simulink model "CTDSM_CIFF_OPAMP_NESTED_CHOPPING"  (R2025b)
settings: Solver=VariableStepAuto  StartTime=0.0  StopTime=0.5  RelTol=1e-3
libraries: fl_lib x19, nesl_utility x8, ee_lib x4, simulink_extras x1, cstblocks x1, dspobslib x1
settings Model: Creator=Hp  LastModifiedBy=k2vas

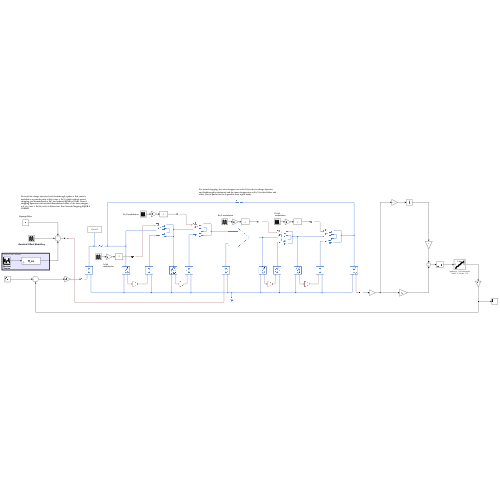
[thumbnail: Simulink's stored preview of the top-level diagram]
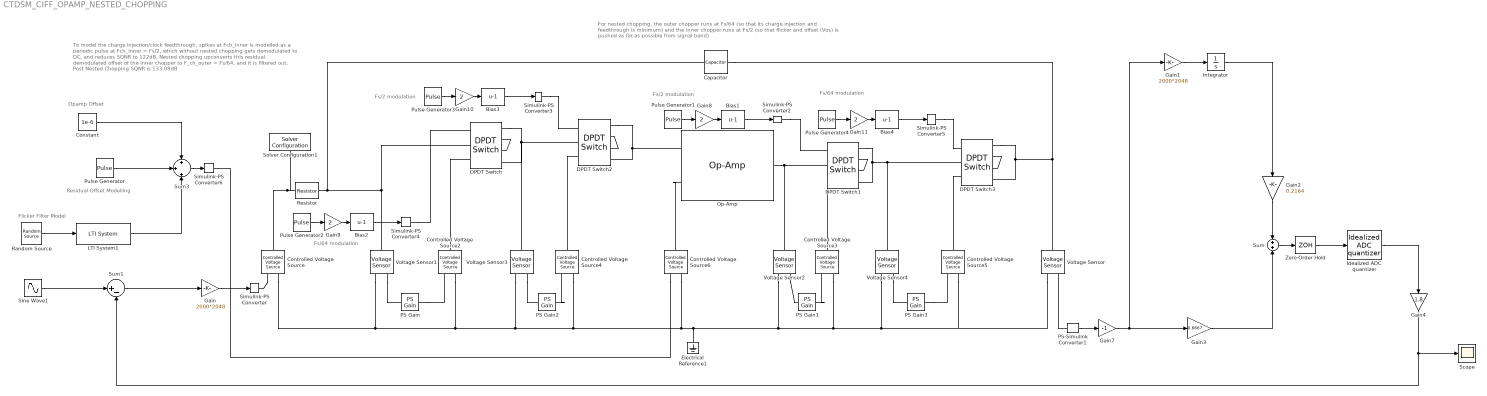
== system CTDSM_CIFF_OPAMP_NESTED_CHOPPING ==
  note: Residual Offset Modelling
  note: Opamp Offset
  note: Fs/2 modulation
  note: Fs/64
      | modulation
  note: Fs/2 modulation
  note: Fs/64
      | modulation
  note: To model the charge injection/clock feedthrough, spikes at Fch_inner is modelled as a periodic pulse at Fch_inner = Fs/2, which without nested chopping gets demodulated to DC, and reduces SQNR to 122dB. Nested chopping upconverts this residual demodulated offset of the inner chopper to F_ch_outer = Fs/64, and it is filtered out. Post Nested Chopping SQNR is 133.09dB
  note: For nested chopping, the outer chopper runs at Fs/64 (so that its charge injection
      | and feedthrough is minimum) and the inner chopper runs at Fs/2 (so that flicker and
      | offset (Vos) is pushed as far as possible from signal band)
  note: Flicker Filter Model
  Bias{1..4} (4 alike) : Bias  Bias=-1  SaturateOnIntegerOverflow=off
  Capacitor : fl_lib/Electrical/Electrical Elements/Capacitor  c=1 F  r=0 Ohm  g=0 1/Ohm  i_specify=off  i_priority=None  i=0 A  i_nominal_specify=off  i_nominal_value=1  i_nominal_unit=A  v_specify=off  v_priority=None  v=0 V  v_nominal_specify=off  v_nominal_value=1  v_nominal_unit=V  vc_specify=off  vc_priority=High  vc=0 V  vc_nominal_specify=off  vc_nominal_value=1  vc_nominal_unit=V
  Constant : Constant  Value=1e-6
  Controlled Voltage Source{,2..6} (6 alike) : fl_lib/Electrical/Electrical Sources/Controlled Voltage Source
  DPDT Switch{,1..3} (4 alike) : ee_lib/Switches & Breakers/DPDT Switch  R_closed=0.01 Ohm  G_open=1e-6 S  Threshold=0.5 V  Width=0 V  model_dynamics=0  t_on=1e-3 s  t_off=1e-3 s  initial_vT=0 V
      settings: InternalSimscapePortConfiguration="{\"Bottom\":[],\"Left\":[{\"id\":\"vT\",\"label\":\"vT\",\"type\":\"input\"},{\"id\":\"p1\",\"label\":\"\",\"type\":\"foundation.electrical.electrical\"},{\"id\":\"p2\",\"label\":\"\",\"type\":\"foundation.electrical.electrical\"}],\"Right\":[{\"id\":\"n11\",\"label\":\"\",\"type\":\"foundation.electrical.electrical\"},{\"id\":\"n12\",\"label\":\"\",\"type\":\"foundation.electrical.electrical\"},{\"id\":\"n21\",\"label\":\"\",\"type\":\"foundation.electrical.electrical\"},{\"id\":\"n22\",\"label\":\"\",\"type\":\"foundation.electrical.electrical\"}],\"Top\":[]}"
  Electrical Reference1 : fl_lib/Electrical/Electrical Elements/Electrical Reference
  Gain : Gain  Gain=2000*2048
  Gain1 : Gain  Gain=2000*2048
  Gain{8..11} (4 alike) : Gain  Gain=2
  Gain2 : Gain  Gain=0.2164
  Gain3 : Gain  Gain=0.6667
  Gain4 : Gain  Gain=1.8
  Gain7 : Gain  Gain=-1
  Idealized ADC quantizer : simulink_extras/Additional Discrete/Idealized ADC quantizer  NumberOfConverterBits=1  Vmin=0  Vmax=1.8  OutputDataType=double  OutputNegativeValues=off
  Integrator : Integrator
  LTI System1 : cstblocks/LTI System  sys=ff_ss  IC=[]  PadeOrder=0
  Op-Amp : fl_lib/Electrical/Electrical Elements/Op-Amp  outI_specify=off  outI_priority=None  outI=0 A  outI_nominal_specify=off  outI_nominal_value=1  outI_nominal_unit=A
  PS Gain{,1..3} (4 alike) : fl_lib/Physical Signals/Functions/PS Gain  gain=-1
  PS-Simulink Converter1 : nesl_utility/PS-Simulink Converter  PhysicalDomain=network_engine_domain  SubClassName=ps_output  LeftPortType=input  RightPortType=output  PseudoPeriodic=off  Frequencies=[]  VectorFormat=inherit  Unit=inherit  AffineConversion=off
  Pulse Generator : DiscretePulseGenerator  PulseType=Time based  Amplitude=2  Period=2/(2000*2048)  PulseWidth=50
  Pulse Generator1 : DiscretePulseGenerator  PulseType=Time based  Period=2/(2000*2048)  PulseWidth=50
  Pulse Generator2 : DiscretePulseGenerator  PulseType=Time based  Period=64/(2048*2000)  PulseWidth=50
  Pulse Generator3 : DiscretePulseGenerator  PulseType=Time based  Period=2/(2048*2000)  PulseWidth=50
  Pulse Generator4 : DiscretePulseGenerator  PulseType=Time based  Period=64/(2048*2000)  PulseWidth=50
  Random Source : dspobslib/Random Source  SrcType=Gaussian  NormMethod=Ziggurat  CltLength=12  MinVal=0  MaxVal=1  MeanVal=0  VarVal=1e-8  RepMode=Not repeatable  rawSeed=1  IsInherit=off  SampMode=Continuous  SampTime=1/(2000*2048)  SampFrame=1  DataType=Double  OutComplex=Real  OutputFrames=off
  Resistor : fl_lib/Electrical/Electrical Elements/Resistor  R=1 Ohm  i_specify=off  i_priority=None  i=0 A  i_nominal_specify=off  i_nominal_value=1  i_nominal_unit=A  v_specify=off  v_priority=None  v=0 V  v_nominal_specify=off  v_nominal_value=1  v_nominal_unit=V
  Scope : Scope
      settings: ActiveDisplayYMinimum=-0.225  ActiveDisplayYMaximum=2.025  DataLoggingVariableName=output_data  DataLoggingSaveFormat=Array
  Simulink-PS Converter{,2..6} (6 alike) : nesl_utility/Simulink-PS Converter  PhysicalDomain=network_engine_domain  SubClassName=ps_input  LeftPortType=input  RightPortType=output  PseudoPeriodic=off  Frequencies=[]  NoiseDistribution=none  NoiseParameters=[]  Unit=1  AffineConversion=off  FilteringAndDerivatives=provide  SimscapeFilterOrder=1  InputFilterTimeConstant=0.001  UdotUserProvided=0
  Sine Wave1 : Sin  Amplitude=0.5  Bias=0.9  Frequency=((2000*1024)*127*2*2*pi)/(32768*32)  SampleTime=0
  Solver Configuration1 : nesl_utility/Solver Configuration  PhysicalDomain=network_engine_domain  SubClassName=solver  LeftPortType=input  RightPortType=generic  Tones=[]  Harmonics=[]  SimulateNoise=off  Profile=off  UseLocalSampling=off  EnableSwitchedLinearOptims=on  FrequencyDomain=off  UseCCode=off  RelTol=0.001  AbsTol=0.001  MinStep=1e-09  ToWorkspace=off  RevertToSquareIcSolve=off  NumHomotopyIterations=100  PhasorMode=off  PhasorModeNumHarmonics=1  ConsistencySolver=NEWTON_XTOL_AFTER_FTOL  IndexReductionMethod=DerivativeReplacement  DoDC=off  ResidualTolerance=1e-09  ConsistencyTolSource=GLOBAL  ConsistencyAbsTol=0.001  ConsistencyRelTol=0.001  ConsistencyTolFactor=0.001  UseLocalSolver=off  LocalSolverChoice=NE_BACKWARD_EULER_ADVANCER  ResolveIndetEquations=on  FunctionEvalNumThread=1  LocalSolverSampleTime=0.001  DoFixedCost=off  MaxNonlinIter=3  MaxModeIter=2  ComputeImpulses=off  ImpulseIterations=2  LinearAlgebra=auto  LinearAlgebraNumThread=0  EquationFormulation=NE_TIME_EF  DelaysMemoryBudget=1024  AutomaticFiltering=on  FilteringTimeConstant=0.001  PartitionStorageMethod=AS_NEEDED  PartitionMemoryBudget=1024  PartitionMethod=ROBUST  MultibodyUseLocalSolver=off  MultibodyLocalSolverChoice=ODE1  MultibodyLocalSolverSampleTime=0.001
  Sum : Sum  Inputs=+|+
  Sum1 : Sum  Inputs=|+-
  Sum3 : Sum  Inputs=+|+|+
  Voltage Sensor{,1..4} (5 alike) : fl_lib/Electrical/Electrical Sensors/Voltage Sensor
  Zero-Order Hold : ZeroOrderHold  SampleTime=1/(2000*1024*2)
  wires:
  Sum1/1 -> Gain/1
  Gain2/1 -> Sum/1
  Gain3/1 -> Sum/2
  PS-Simulink Converter1/1 -> Gain7/1
  Zero-Order Hold/1 -> Idealized ADC quantizer/1
  Idealized ADC quantizer/1 -> Gain4/1
  Gain1/1 -> Integrator/1
  Gain4/1 -> Sum1/2, Scope/1
  Sum/1 -> Zero-Order Hold/1
  Sine Wave1/1 -> Sum1/1
  Gain7/1 -> Gain3/1, Gain1/1
  Bias1/1 -> Simulink-PS Converter2/1
  Pulse Generator1/1 -> Gain8/1
  Gain8/1 -> Bias1/1
  Pulse Generator2/1 -> Gain9/1
  Bias2/1 -> Simulink-PS Converter4/1
  Gain9/1 -> Bias2/1
  Bias3/1 -> Simulink-PS Converter3/1
  Pulse Generator3/1 -> Gain10/1
  Gain10/1 -> Bias3/1
  Pulse Generator4/1 -> Gain11/1
  Bias4/1 -> Simulink-PS Converter5/1
  Gain11/1 -> Bias4/1
  Sum3/1 -> Simulink-PS Converter6/1
  Pulse Generator/1 -> Sum3/2
  Constant/1 -> Sum3/1
  LTI System1/1 -> Sum3/3
  Integrator/1 -> Gain2/1
  Gain/1 -> Simulink-PS Converter/1
  Random Source/1 -> LTI System1/1
  connections:
  Controlled Voltage Source/LConn1 -- Solver Configuration1/RConn1 -- Resistor/LConn1
  PS-Simulink Converter1/LConn1 -- Voltage Sensor/RConn1
  Controlled Voltage Source/RConn1 -- Simulink-PS Converter/RConn1
  DPDT Switch/RConn1 -- Voltage Sensor3/LConn1 -- DPDT Switch/RConn4 -- DPDT Switch2/LConn2
  Op-Amp/RConn1 -- Voltage Sensor2/LConn1 -- DPDT Switch1/LConn2
  DPDT Switch/RConn2 -- DPDT Switch/RConn3
  Simulink-PS Converter4/RConn1 -- DPDT Switch/LConn1
  Simulink-PS Converter2/RConn1 -- DPDT Switch1/LConn1
  Voltage Sensor1/RConn1 -- PS Gain/LConn1
  PS Gain/RConn1 -- Controlled Voltage Source2/RConn1
  Voltage Sensor2/RConn1 -- PS Gain1/LConn1
  PS Gain1/RConn1 -- Controlled Voltage Source3/RConn1
  Controlled Voltage Source3/LConn1 -- DPDT Switch1/LConn3
  DPDT Switch1/RConn2 -- DPDT Switch1/RConn3
  Voltage Sensor1/RConn2 -- Controlled Voltage Source2/RConn2 -- Controlled Voltage Source4/RConn2 -- Controlled Voltage Source6/RConn2 -- Voltage Sensor/RConn2 -- Controlled Voltage Source5/RConn2 -- Voltage Sensor4/RConn2 -- Controlled Voltage Source3/RConn2 -- Voltage Sensor2/RConn2 -- Electrical Reference1/LConn1 -- Voltage Sensor3/RConn2 -- Controlled Voltage Source/RConn2
  DPDT Switch2/RConn3 -- DPDT Switch2/RConn2
  DPDT Switch2/RConn1 -- DPDT Switch2/RConn4 -- Op-Amp/LConn2
  Voltage Sensor3/RConn1 -- PS Gain2/LConn1
  Controlled Voltage Source4/LConn1 -- DPDT Switch2/LConn3
  PS Gain2/RConn1 -- Controlled Voltage Source4/RConn1
  Simulink-PS Converter3/RConn1 -- DPDT Switch2/LConn1
  DPDT Switch3/RConn2 -- DPDT Switch3/RConn3
  PS Gain3/RConn1 -- Controlled Voltage Source5/RConn1
  Voltage Sensor4/RConn1 -- PS Gain3/LConn1
  Simulink-PS Converter5/RConn1 -- DPDT Switch3/LConn1
  DPDT Switch1/RConn1 -- DPDT Switch3/LConn2 -- Voltage Sensor4/LConn1 -- DPDT Switch1/RConn4
  Voltage Sensor1/LConn1 -- Resistor/RConn1 -- Capacitor/LConn1 -- DPDT Switch/LConn2
  DPDT Switch3/LConn3 -- Controlled Voltage Source5/LConn1
  DPDT Switch/LConn3 -- Controlled Voltage Source2/LConn1
  Op-Amp/LConn1 -- Controlled Voltage Source6/LConn1
  Controlled Voltage Source6/RConn1 -- Simulink-PS Converter6/RConn1
  DPDT Switch3/RConn1 -- DPDT Switch3/RConn4 -- Voltage Sensor/LConn1 -- Capacitor/RConn1
